simulink model "cholSFun"  (R2015b)
settings: Solver=FixedStepDiscrete  StartTime=0.0  StopTime=10.0  FixedStep=0.001  RelTol=1e-3
values from neighbouring files (symbols this model uses):
  W = chol(P)    [initSim.m]
  x = xScale*(rand(N, 1) - 0.5).*(10.^((rand(N, 1) - 0.5)))    [initSim.m]    (also in testDowndateAgainstCholupdate.m)
settings Model: Creator=niermeyer  LastModifiedBy=niermeyer

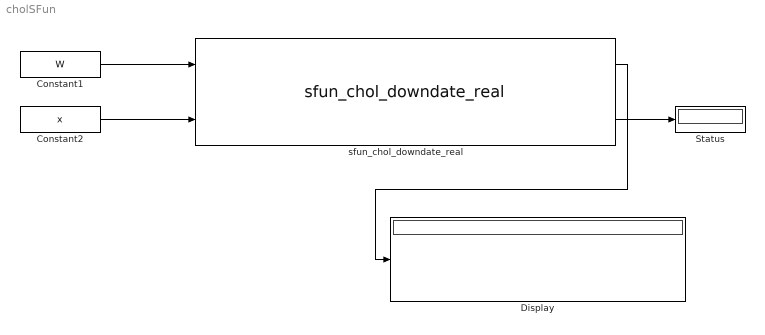
== system cholSFun ==
  Constant1 : Constant  Value=W
  Constant2 : Constant  Value=x
  Display : Display
  Status : Display
  sfun_chol_downdate_real : S-Function  FunctionName=sfun_chol_downdate_real  Parameters=SParameter1  SFunctionDeploymentMode=off  EnableBusSupport=off  mask(Legacy Function){SFunctionSpec=sFunWrapper(double y1[size(u1,1)][size(u1,2)], uint32 p1[1], double u1[][], double u2[]), SParameter1=4, ShowSpec=on}
      mask prompts: SParameter1 "P1:"; ShowSpec "Display function specification"
      mask help:
      | This block allows you to call the legacy functions specified by the following Legacy Code Tool definition:
      | def.SFunctionName = 'sfun_chol_downdate_real';
      | def.OutputFcnSpec = 'sFunWrapper(double y1[size(u1,1)][size(u1,2)], uint32 p1[1], double u1[][], double u2[])';
      | def.HeaderFiles = {'math.h', 'mex.h', 'matrix.h'};
      | def.SourceFiles = {'CholeskyDowndateReal.c'};
      mask Help: <p>This block was generated automatically by the Legacy Code Tool. For detailed help on this tool, call<a href="matlab:legacy_code('help')"> legacy_code('help')</a>.</p>
      mask Callback ShowSpec:
      | if strcmp(get_param(gcbh, 'ShowSpec'), 'on')
      |   set_param(gcbh, 'MaskDisplay', sprintf('fprintf(''%s'');', get_param(gcbh, 'SFunctionSpec')));
      | else
      |   set_param(gcbh, 'MaskDisplay', sprintf('fprintf(''%s'');', get_param(gcbh, 'FunctionName')));
      | end
      mask Display: fprintf('sFunWrapper(double y1[size(u1,1)][size(u1,2)], uint32 p1[1], double u1[][], double u2[])');
  wires:
  Constant2/1 -> sfun_chol_downdate_real/2
  sfun_chol_downdate_real/1 -> Display/1
  sfun_chol_downdate_real/2 -> Status/1
  Constant1/1 -> sfun_chol_downdate_real/1
